simulink model "tcs2"  (R2024b)
settings: Solver=ode45  StartTime=0.0  StopTime=10  RelTol=1e-3
InitFcn:
  | Cte_Traction
values from neighbouring files (symbols this model uses):
  b = 0.00005    (= 5e-05)    [Cte_Traction.m]
  g = 9.81    [Cte_TP_ABS_CHERIF.m]    (also in Cte_Traction.m)
  GR = 1    [Cte_Traction.m]
  J = 0.5    [Cte_TP_ABS_CHERIF.m]    (also in Cte_Traction.m)
  Kb = 0.7    [Cte_Traction.m]
  Kd = 0    [Cte_TP_ABS_CHERIF.m]
  Km = 10    [Cte_TP_ABS_CHERIF.m]    (also in Cte_Traction.m = 0.7)
  L = d_avant + d_arriere    (= 3)    [Cte_TP_ABS_CHERIF.m]    (also in Cte_Traction.m = 0.0005)
  m = 1000    [Cte_TP_ABS_CHERIF.m]    (also in Cte_Traction.m = 1500)
  Q = 0.25    [Cte_Traction.m]
  R = 0.01    [Cte_Traction.m]
  Rw = 0.3    [Cte_Traction.m]
settings Model: Creator=enzoc  LastModifiedBy=enzoc

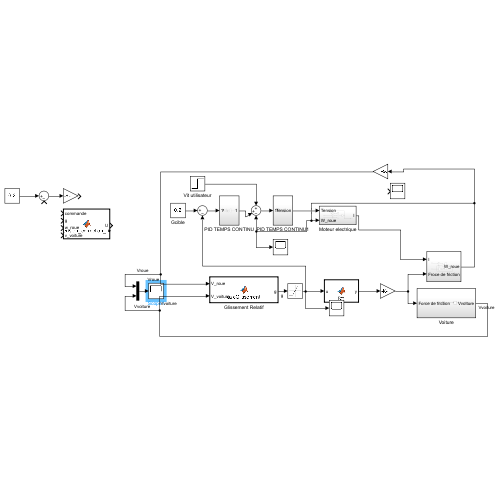
[thumbnail: Simulink's stored preview of the top-level diagram]
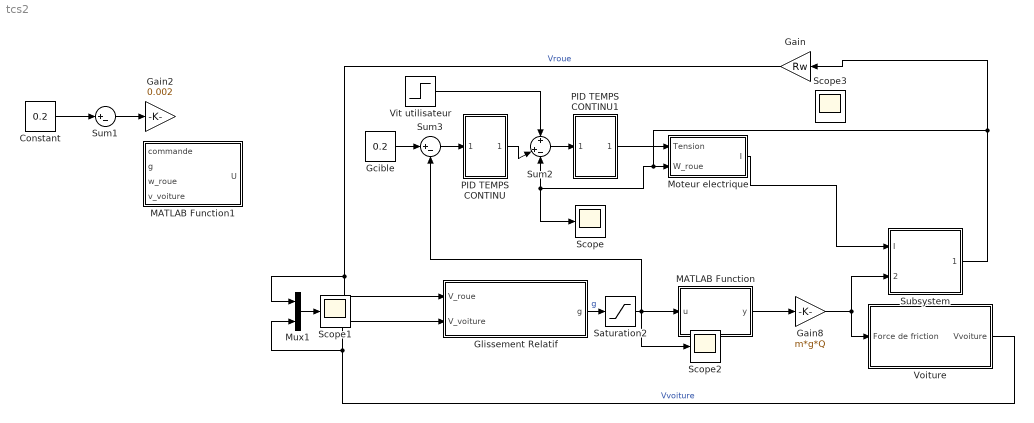
== system tcs2 ==
  Constant : Constant  Value=0.2
  Gain : Gain  Gain=Rw
  Gain2 : Gain  Gain=0.002
  Gain8 : Gain  Gain=m*g*Q
  Gcible : Constant  Value=0.2
  Glissement Relatif : MATLAB Function  TreatAsAtomicUnit=on
  MATLAB Function : MATLAB Function  TreatAsAtomicUnit=on
  MATLAB Function1 : MATLAB Function  TreatAsAtomicUnit=on
  Moteur electrique : Subsystem
  Mux1 : Mux  Inputs=2
  PID TEMPS CONTINU : Subsystem
  PID TEMPS CONTINU1 : Subsystem
  Saturation2 : Saturate  UpperLimit=1  LowerLimit=-1
  Scope{,1..3} (4 alike) : Scope
  Subsystem : Subsystem
  Sum1 : Sum  Inputs=|+-
  Sum2 : Sum  Inputs=+|+-
  Sum3 : Sum  Inputs=|+-
  Vit utilisateur : Step  Time=400  SampleTime=0
  Voiture : Subsystem
  wires:
  Glissement Relatif/1(g) -> Saturation2/1  "g"
  MATLAB Function/1(y) -> Gain8/1
  Gain8/1 -> Voiture/1(Force de friction), Subsystem/2(Froce de friction)
  Voiture/1(Vvoiture) -> Mux1/2, Glissement Relatif/2(V_voiture)  "Vvoiture"
  Moteur electrique/1(I) -> Subsystem/1(I)
  Subsystem/1(W_roue) -> Gain/1, Moteur electrique/2(W_roue), Scope/1, Sum2/3
  Gain/1 -> Mux1/1, Glissement Relatif/1(V_roue)  "Vroue"
  Mux1/1 -> Scope1/1
  Sum1/1 -> Gain2/1
  Constant/1 -> Sum1/1
  Saturation2/1 -> Sum3/2, MATLAB Function/1(u), Scope2/1
  Sum2/1 -> PID TEMPS CONTINU1/1(In1)
  Gcible/1 -> Sum3/1
  Sum3/1 -> PID TEMPS CONTINU/1(In1)
  Vit utilisateur/1 -> Sum2/1
  PID TEMPS CONTINU/1(Out1) -> Sum2/2
  PID TEMPS CONTINU1/1(Tension) -> Moteur electrique/1(Tension)

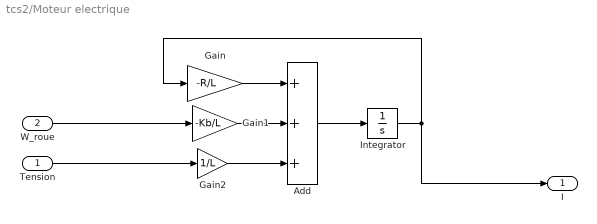
== system tcs2/Moteur electrique ==
  Tension : Inport
  W_roue : Inport  Port=2
  Add : Sum  Inputs=+++
  Gain : Gain  Gain=-R/L
  Gain1 : Gain  Gain=-Kb/L
  Gain2 : Gain  Gain=1/L
  Integrator : Integrator
  I : Outport
  wires:
  Tension/1 -> Gain2/1
  Integrator/1 -> I/1, Gain/1
  Gain2/1 -> Add/3
  Add/1 -> Integrator/1
  Gain/1 -> Add/1
  Gain1/1 -> Add/2
  W_roue/1 -> Gain1/1

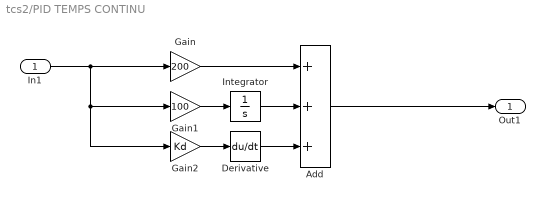
== system tcs2/PID TEMPS CONTINU ==
  In1 : Inport
  Add : Sum  Inputs=+++
  Derivative : Derivative
  Gain : Gain  Gain=200
  Gain1 : Gain  Gain=100
  Gain2 : Gain  Gain=Kd
  Integrator : Integrator
  Out1 : Outport
  wires:
  Derivative/1 -> Add/3
  Add/1 -> Out1/1
  In1/1 -> Gain2/1, Gain1/1, Gain/1
  Gain/1 -> Add/1
  Gain2/1 -> Derivative/1
  Integrator/1 -> Add/2
  Gain1/1 -> Integrator/1

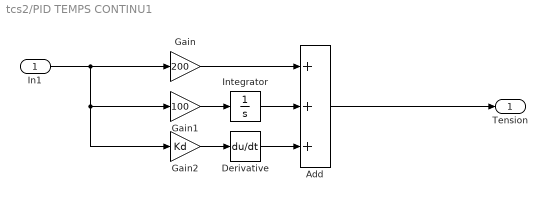
== system tcs2/PID TEMPS CONTINU1 ==
  In1 : Inport
  Add : Sum  Inputs=+++
  Derivative : Derivative
  Gain : Gain  Gain=200
  Gain1 : Gain  Gain=100
  Gain2 : Gain  Gain=Kd
  Integrator : Integrator
  Tension : Outport
  wires:
  Derivative/1 -> Add/3
  Add/1 -> Tension/1
  In1/1 -> Gain2/1, Gain1/1, Gain/1
  Gain/1 -> Add/1
  Gain2/1 -> Derivative/1
  Integrator/1 -> Add/2
  Gain1/1 -> Integrator/1

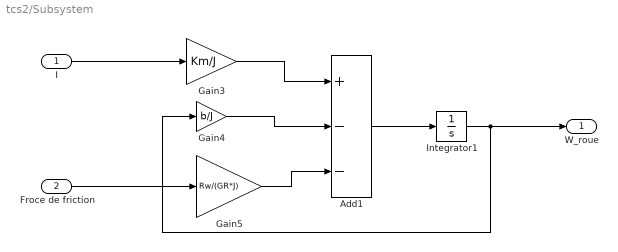
== system tcs2/Subsystem ==
  I : Inport
  Froce de friction : Inport  Port=2
  Add1 : Sum  Inputs=+--
  Gain3 : Gain  Gain=Km/J
  Gain4 : Gain  Gain=b/J
  Gain5 : Gain  Gain=Rw/(GR*J)
  Integrator1 : Integrator
  W_roue : Outport
  wires:
  Froce de friction/1 -> Gain5/1
  Add1/1 -> Integrator1/1
  Integrator1/1 -> Gain4/1, W_roue/1
  Gain5/1 -> Add1/3
  Gain4/1 -> Add1/2
  I/1 -> Gain3/1
  Gain3/1 -> Add1/1

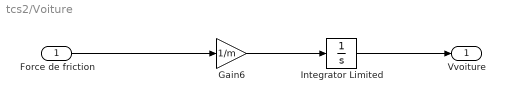
== system tcs2/Voiture ==
  Force de friction : Inport
  Gain6 : Gain  Gain=1/m
  Integrator Limited : Integrator  LimitOutput=on  UpperSaturationLimit=+inf  LowerSaturationLimit=0
  Vvoiture : Outport
  wires:
  Gain6/1 -> Integrator Limited/1
  Integrator Limited/1 -> Vvoiture/1
  Force de friction/1 -> Gain6/1

== matlab function tcs2/Glissement Relatif ==
  data: V_roue input; V_voiture input; g output
function g = calcGlissement(V_roue, V_voiture)
    g = (V_roue-V_voiture)/(abs(V_voiture)+0.001);
end

== matlab function tcs2/MATLAB Function ==
  data: u input; y output
function y = fcn(u)

y = u;

== matlab function tcs2/MATLAB Function1 ==
  settings: updateMethod=DISCRETE
  data: commande input; U output; g input; w_roue input; v_voiture input
function U = calc_tension_correction_fixed_g(commande, g, w_roue, v_voiture)
    % calc_tension_correction_fixed_g : Corrige la tension pour maintenir g = 0.005 avec contrôle PID
    % Entrées :
    %   commande  : Commande utilisateur (valeur entre 0 et 1)
    %   g         : Glissement actuel (valeur entre 0 et 1)
    %   w_roue    : Vitesse angulaire actuelle de la roue (en rad/s)
    %   v_voiture : Vitesse cible du véhicule (en m/s)
    % Sortie :
    %   U         : Tension corrigée à appliquer au moteur (en Volts)

    % Paramètres physiques
    Rw = 0.3;          % Rayon de la roue (m)
    Vmax = 400;        % Tension maximale (Volts)
    GR = 9;            % Rapport de réduction
    g_cible = 0.005;   % Glissement cible (réduit pour une meilleure adhérence)

    % Gains du contrôleur PID
    K_p = 150;         % Gain proportionnel (augmenté pour une correction plus rapide)
    K_i = 100;         % Gain intégral (augmenté pour réduire l'erreur résiduelle)
    K_d = 10;          % Gain dérivé (inchangé pour limiter les oscillations)

    % Constantes du filtre passe-bas
    alpha = 0.85;      % Coefficient du filtre (légèrement réduit pour accélérer la réponse)

    % Variables persistantes pour conserver les valeurs entre appels
    persistent integral_glissement prev_erreur_glissement dt U_previous
    if isempty(integral_glissement)
        integral_glissement = 0;   % Initialisation de l'intégrale du glissement
        prev_erreur_glissement = 0; % Initialisation de l'erreur précédente
        dt = 0.01;                % Pas de temps (10 ms)
        U_previous = 0;           % Initialisation de la tension précédente
    end

    % Étape 1 : Tension initiale basée sur la commande utilisateur
    U = commande * Vmax;

    % Étape 2 : Correction pour maintenir g = g_cible si le glissement dépasse la cible
    if g > g_cible
        % Calcul de l'erreur de glissement
        erreur_glissement = g_cible - g;

        % Mise à jour de l'intégrale du glissement
        integral_glissement = integral_glissement + erreur_glissement * dt;

        % Calcul de la dérivée de l'erreur
        deriv_erreur_glissement = (erreur_glissement - prev_erreur_glissement) / dt;

        % Mise à jour de l'erreur précédente
        prev_erreur_glissement = erreur_glissement;

        % Calcul de la correction PID
        correction_glissement = K_p * erreur_glissement + K_i * integral_glissement + K_d * deriv_erreur_glissement;

        % Limitation de la correction pour éviter une sur-correction
        correction_glissement = max(-Vmax / 2, min(Vmax / 2, correction_glissement));

        % Ajustement de la tension
        U = U + correction_glissement;
    end

    % Étape 3 : Application du filtre passe-bas
    U = alpha * U_previous + (1 - alpha) * U;

    % Mise à jour de la tension précédente
    U_previous = U;

    % Étape 4 : Limitation de la tension
    U = max(0, min(Vmax, U)); % Assure que la tension reste dans la plage [0, Vmax])
end
